simulink model "model_raspuns"  (R2023b)
settings: Solver=VariableStepAuto  StartTime=0.0  StopTime=30  RelTol=1e-3
values from neighbouring files (symbols this model uses):
  ustar = zeros(10, 1)    [Modelul2_Pendulul_elastic.m]
undefined symbols (not defined in the file or in its folder): A_lin, B_lin, C_lin, D_lin, xstar, ystar
settings Model: Creator=gabri  LastModifiedBy=gabri

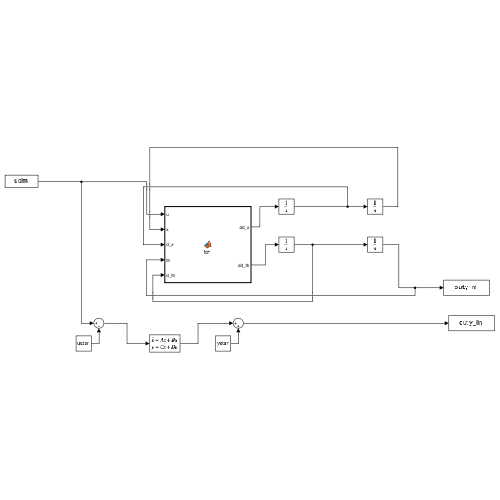
[thumbnail: Simulink's stored preview of the top-level diagram]
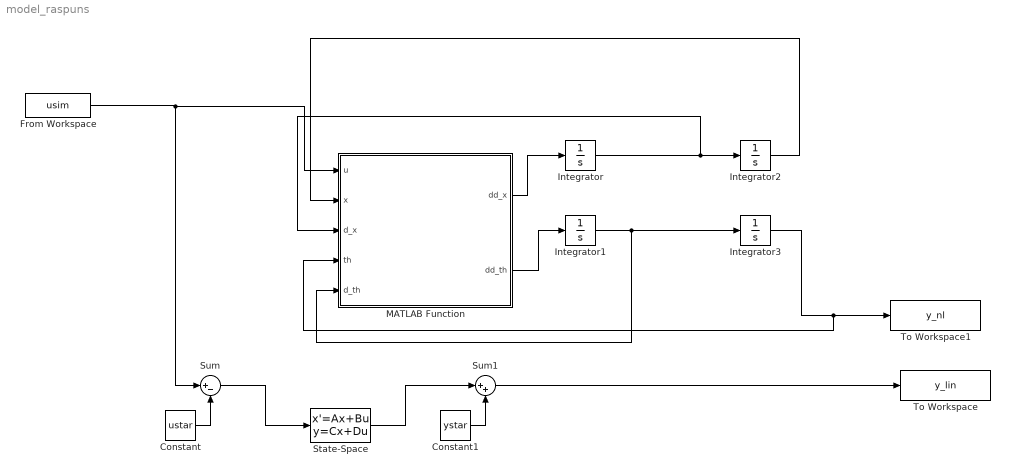
== system model_raspuns ==
  Constant : Constant  Value=ustar
  Constant1 : Constant  Value=ystar
  From Workspace : FromWorkspace  VariableName=usim
  Integrator{,1..3} (4 alike) : Integrator
  MATLAB Function : MATLAB Function  TreatAsAtomicUnit=on
  State-Space : StateSpace  A=A_lin  B=B_lin  C=C_lin  D=D_lin  InitialCondition=-xstar
  Sum : Sum  Inputs=|+-
  Sum1 : Sum  Inputs=|++
  To Workspace : ToWorkspace  VariableName=y_lin  SaveFormat=Timeseries  SampleTime=-1
  To Workspace1 : ToWorkspace  VariableName=y_nl  SaveFormat=Timeseries  SampleTime=-1
      settings: Save2DSignal=2-D array (concatenate along first dimension)
  wires:
  Integrator2/1 -> MATLAB Function/2(x)
  From Workspace/1 -> Sum/1, MATLAB Function/1(u)
  Integrator/1 -> MATLAB Function/3(d_x), Integrator2/1
  MATLAB Function/1(dd_x) -> Integrator/1
  MATLAB Function/2(dd_th) -> Integrator1/1
  Integrator1/1 -> Integrator3/1, MATLAB Function/5(d_th)
  Integrator3/1 -> MATLAB Function/4(th), To Workspace1/1
  Constant/1 -> Sum/2
  Sum1/1 -> To Workspace/1
  Constant1/1 -> Sum1/2
  Sum/1 -> State-Space/1
  State-Space/1 -> Sum1/1

== matlab function model_raspuns/MATLAB Function ==
  data: dd_x output; u input; dd_th output; x input; d_x input; th input; d_th input
function [dd_x, dd_th] = fcn(u, x, d_x, th, d_th)

l0 = 2.42;
m = 4.53;
k = 3.21;
fact = 0.71;
g = 9.81;

    %Ecuatiile
    dd_x = (l0 + x) * (d_th) * (d_th) - ((k * x) / m) + g * cos(th) - fact * d_x;
    dd_th = -(g/(l0+x)*sin(th))-(2*d_x/(l0+x))*d_th - fact*d_th + 1/(m*(l0+x)*(l0+x))*u;

end
